simulink model "satellite_sim_old"  (R2018b)
settings: Solver=ode45  StartTime=0.0  StopTime=200  RelTol=1e-3  EnableMultiTasking=on
InitFcn:
  | addpath ./..
  | satelliteParam
  | satelliteParamHW11
undefined symbols (not defined in the file): P, satellite_animation, satellite_ctrl
settings Model: Creator=beard  LastModifiedBy=beard
settings DataIOCC: LimitDataPoints=on  SaveFormat=Array  SignalLoggingSaveFormat=ModelDataLogs
settings OptimizationCC: ExpressionDepthLimit=2147483647  InitFltsAndDblsToZero=on  LifeSpan=inf
settings DebuggingCC: UnderspecifiedInitializationDetection=Classic  MergeDetectMultiDrivingBlocksExec=none  SolverPrmCheckMsg=warning  FcnCallInpInsideContextMsg=warning  StateNameClashWarn=warning  SFUnexpectedBacktrackingDiag=warning  SFNoUnconditionalDefaultTransitionDiag=warning  SFExecutionAtInitializationDiag=none
settings HardwareCC: ProdBitPerPointer=32  ProdBitPerSizeT=32  ProdBitPerPtrDiffT=32  ProdLargestAtomicFloat=None  ProdIntDivRoundTo=Undefined  ProdEndianess=Unspecified  ProdWordSize=32  ProdHWDeviceType=32-bit Generic
settings ModelReferenceCC: PropagateSignalLabelsOutOfModel=off
settings SFSimCC: SimUseLocalCustomCode=off
settings RTWCC: RTWUseLocalCustomCode=off
settings CodeAppCC: StateflowObjectComments=on
settings GRTTargetCC: TargetLangStandard=C89/C90 (ANSI)  GeneratePreprocessorConditionals=Disable all  CombineOutputUpdateFcns=off  GRTInterface=on
settings ConfigComp: CovMetricSettings=dw  CovHtmlReporting=on  CovSaveCumulativeToWorkspaceVar=on  CovSaveSingleToWorkspaceVar=on  CovExternalEMLEnable=off

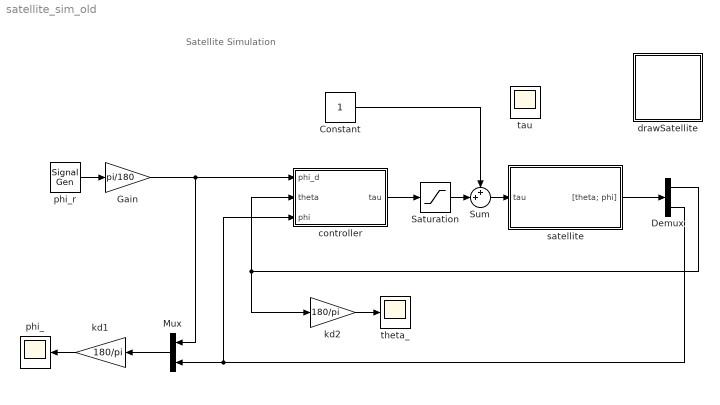
== system satellite_sim_old ==
  note: Satellite Simulation
  Constant : Constant
  Demux : Demux  Outputs=2
  Gain : Gain  Gain=pi/180
  Mux : Mux  Inputs=2
  Saturation : Saturate  UpperLimit=P.taumax  LowerLimit=-P.taumax
  Sum : Sum  Inputs=++|
  controller : Subsystem
  drawSatellite : Subsystem
      mask Display: image(imread('tv.jpg'))
  kd1 : Gain  Gain=180/pi
  kd2 : Gain  Gain=180/pi
  phi_ : Scope
  phi_r : SignalGenerator  WaveForm=square  Amplitude=15  Frequency=.02
  satellite : Subsystem
  tau : Scope
  theta_ : Scope
  wires:
  satellite/1("[theta; phi]") -> Demux/1
  phi_r/1 -> Gain/1
  controller/1(tau) -> Saturation/1
  Demux/1 -> kd2/1, controller/2(theta)
  Demux/2 -> Mux/2, controller/3(phi)
  Gain/1 -> Mux/1, controller/1(phi_d)
  kd2/1 -> theta_/1
  Mux/1 -> kd1/1
  kd1/1 -> phi_/1
  Saturation/1 -> Sum/2
  Sum/1 -> satellite/1(tau)
  Constant/1 -> Sum/1

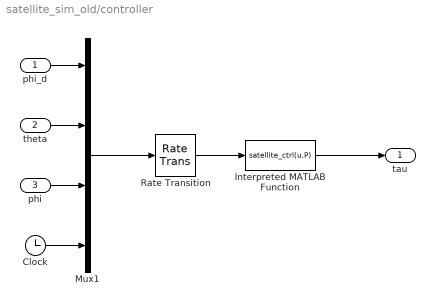
== system satellite_sim_old/controller ==
  phi_d : Inport
  theta : Inport  Port=2
  phi : Inport  Port=3
  Clock : Clock
  Interpreted MATLAB Function : MATLABFcn  MATLABFcn=satellite_ctrl(u,P)  OutputDimensions=1
  Mux1 : Mux
  Rate Transition : RateTransition  OutPortSampleTime=P.Ts
  tau : Outport
  wires:
  Mux1/1 -> Rate Transition/1
  phi_d/1 -> Mux1/1
  Interpreted MATLAB Function/1 -> tau/1
  Clock/1 -> Mux1/4
  Rate Transition/1 -> Interpreted MATLAB Function/1
  phi/1 -> Mux1/3
  theta/1 -> Mux1/2

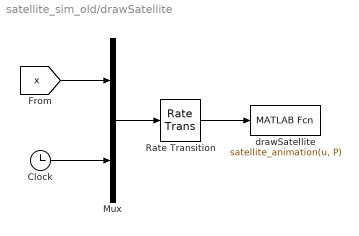
== system satellite_sim_old/drawSatellite ==
  Clock : Clock
  Mux : Mux  Inputs=2
  Rate Transition : RateTransition  OutPortSampleTime=P.t_plot
  drawSatellite : MATLABFcn  MATLABFcn=satellite_animation(u, P)  OutputDimensions=0
  wires:
  Mux/1 -> Rate Transition/1
  [x] -> Mux/1
  Clock/1 -> Mux/2
  Rate Transition/1 -> drawSatellite/1

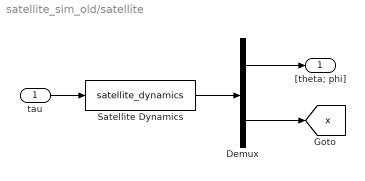
== system satellite_sim_old/satellite ==
  tau : Inport
  Demux : Demux  Outputs=[2;4]
  Satellite Dynamics : S-Function  FunctionName=satellite_dynamics  Parameters=P  SFunctionDeploymentMode=off  EnableBusSupport=off
  "[theta; phi]" : Outport
  tag scope: x=global
  wires:
  tau/1 -> Satellite Dynamics/1
  Satellite Dynamics/1 -> Demux/1
  Demux/1 -> "[theta; phi]"/1
  Demux/2 -> [x]
